simulink model "Hardmon_Model"  (R2023b)
settings: Solver=FixedStepDiscrete  StartTime=0.0  StopTime=10  RelTol=1e-3
libraries: msbUtilities x1
settings Model: Creator=heyka  LastModifiedBy=nickj
settings DataIOCC: ExternalInput=test_temp.getElement('Temp 1'),test_temp.getElement('Temp 2')  LoadExternalInput=on
settings OptimizationCC: DefaultParameterBehavior=Inlined  EnhancedBackFolding=on  PassReuseOutputArgsAs=Individual arguments  ZeroExternalMemoryAtStartup=off  ZeroInternalMemoryAtStartup=off  OptimizeBlockOrder=speed  DifferentSizesBufferReuse=on  OptimizationCustomize=off  EfficientTunableParamExpr=on
settings DebuggingCC: SolverPrmCheckMsg=warning  ParameterTunabilityLossMsg=error  StateNameClashWarn=warning
settings HardwareCC: ProdBitPerInt=16  ProdBitPerPointer=16  ProdBitPerSizeT=16  ProdBitPerPtrDiffT=16  ProdLargestAtomicFloat=None  ProdWordSize=16  ProdHWDeviceType=STMicroelectronics->ST10/Super10
settings SFSimCC: MATLABDynamicMemAlloc=off  SimTargetLang=C++
settings RTWCC: Description=Embedded Coder  SystemTargetFile=ert.tlc  GenCodeOnly=on  TemplateMakefile=ert_default_tmf  Toolchain=MinGW64 | gmake (64-bit Windows)  BuildConfiguration=Faster Runs  PortableWordSizes=on  DataTypeReplacement=CDataTypesFixedWidth  TargetLang=C++
settings CodeAppCC: ForceParamTrailComments=on  IgnoreCustomStorageClasses=off  OperatorAnnotations=on  SimulinkDataObjDesc=on  SFDataObjDesc=on  MATLABFcnDesc=on  InsertBlockDesc=on  StateflowObjectComments=on  InlinedPrmAccess=Macros
settings ERTTargetCC: TargetLangStandard=C++11 (ISO)  GenerateSampleERTMain=on  CodeInterfacePackaging=C++ class  SupportNonFinite=off  SupportComplex=off  CastingMode=Standards  ArrayLayout=Row-major  InlinedParameterPlacement=NonHierarchical  RootIOFormat=Structure reference  ERTCustomFileTemplate=example_file_process.tlc  ERTFilePackagingFormat=Compact  SuppressUnreachableDefaultCases=off  IndentSize=4  MaxIdInt64=INT64_MAX  MinIdInt64=INT64_MIN  MaxIdUint64=UINT64_MAX  MaxIdInt32=INT32_MAX  MinIdInt32=INT32_MIN  MaxIdUint32=UINT32_MAX  MaxIdInt16=INT16_MAX  MinIdInt16=INT16_MIN  MaxIdUint16=UINT16_MAX  MaxIdInt8=INT8_MAX  MinIdInt8=INT8_MIN  MaxIdUint8=UINT8_MAX

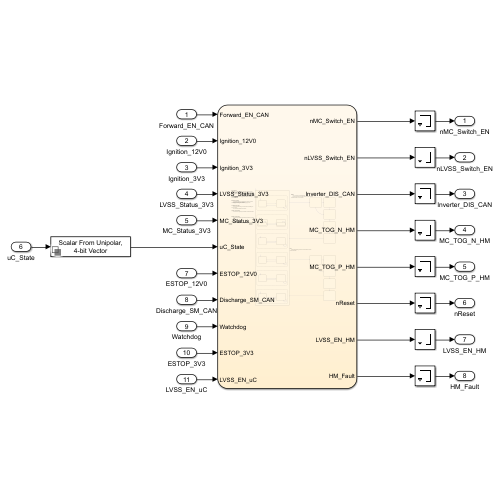
[thumbnail: Simulink's stored preview of the top-level diagram]
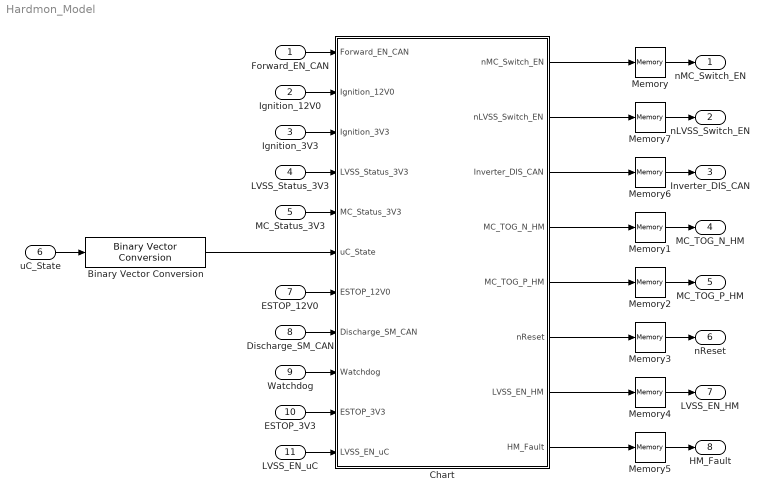
== system Hardmon_Model ==
  Forward_EN_CAN : Inport  OutDataTypeStr=boolean
  Ignition_12V0 : Inport  Port=2  OutDataTypeStr=boolean
  Ignition_3V3 : Inport  Port=3  OutDataTypeStr=boolean
  LVSS_Status_3V3 : Inport  Port=4  OutDataTypeStr=boolean
  MC_Status_3V3 : Inport  Port=5  OutDataTypeStr=boolean
  uC_State : Inport  Port=6  OutDataTypeStr=uint8  PortDimensions=4
  ESTOP_12V0 : Inport  Port=7  OutDataTypeStr=boolean
  Discharge_SM_CAN : Inport  Port=8  OutDataTypeStr=uint8
  Watchdog : Inport  Port=9  OutDataTypeStr=boolean
  ESTOP_3V3 : Inport  Port=10  OutDataTypeStr=boolean
  LVSS_EN_uC : Inport  Port=11  OutDataTypeStr=boolean
  Binary Vector Conversion : msbUtilities/Binary Vector Conversion  LabelModeActiveChoice=From Unipolar  Convert=Binary-coded vector to scalar  Encoding=Unipolar (magnitude)  InputLength=4  InputReverse=LSB at index 1  OutputLength=4  OutputReverse=LSB at index 1  DataType=uint8
  Chart : Stateflow chart  TreatAsAtomicUnit=on
      settings: PortSchema="{\"entries\":[{\"content\":{\"sides\":[{\"content\":{\"connectorIds\":[\"In1\",\"In2\",\"In3\",\"In4\",\"In5\",\"In6\",\"In7\",\"In8\",\"In9\",\"In10\",\"In11\"]},\"type\":\"ConnectorPlacement.EquallySpacedRectSide\",\"uuid\":\"6d1a41ef-67e8-41d6-9adb-1761831f6d0e\"},{\"content\":{\"connectorIds\":[\"Out1\",\"Out8\",\"Out2\",\"Out3\",\"Out4\",\"Out5\",\"Out6\",\"Out7\"],\"side\":\"RIGHT\"},\"type\":\"ConnectorPlacement.EquallySpacedRectSide\",\"uuid\":\"1c1f5b1f-9a19-48ee-ac61-8a13c1cfd4a8\"},{\"content\":{\"side\":\"TOP\"},\"type\":\"ConnectorPlacement.EquallySpacedRectSide\",\"uuid\":\"7f8ec887-50f7-4fb3-9eed-5aef04cf2afb\"}]},\"type\":\"ConnectorPlacement.EquallySpacedConnector\",\"uuid\":\"822c8876-1e52-4482-83f3-7114ae95ed93\"}],\"packageUris\":[\"http://schema.mathworks.com/mf0/Connector/R2020b\"],\"version\":\"1.0\"}"
  Memory{,1..7} (8 alike) : Memory
  nMC_Switch_EN : Outport  OutDataTypeStr=boolean
  nLVSS_Switch_EN : Outport  Port=2  OutDataTypeStr=boolean
  Inverter_DIS_CAN : Outport  Port=3  OutDataTypeStr=boolean
  MC_TOG_N_HM : Outport  Port=4  OutDataTypeStr=boolean
  MC_TOG_P_HM : Outport  Port=5  OutDataTypeStr=boolean
  nReset : Outport  Port=6  OutDataTypeStr=boolean
  LVSS_EN_HM : Outport  Port=7  OutDataTypeStr=boolean
  HM_Fault : Outport  Port=8  OutDataTypeStr=boolean
  wires:
  Chart/7(HM_Fault) -> Memory5/1
  uC_State/1 -> Binary Vector Conversion/1
  Forward_EN_CAN/1 -> Chart/1(Forward_EN_CAN)
  Binary Vector Conversion/1 -> Chart/6(uC_State)
  LVSS_Status_3V3/1 -> Chart/4(LVSS_Status_3V3)
  Chart/6(LVSS_EN_HM) -> Memory4/1
  Ignition_12V0/1 -> Chart/2(Ignition_12V0)
  Ignition_3V3/1 -> Chart/3(Ignition_3V3)
  MC_Status_3V3/1 -> Chart/5(MC_Status_3V3)
  ESTOP_12V0/1 -> Chart/7(ESTOP_12V0)
  Discharge_SM_CAN/1 -> Chart/8(Discharge_SM_CAN)
  Watchdog/1 -> Chart/9(Watchdog)
  ESTOP_3V3/1 -> Chart/10(ESTOP_3V3)
  LVSS_EN_uC/1 -> Chart/11(LVSS_EN_uC)
  Chart/1(nMC_Switch_EN) -> Memory/1
  Chart/2(Inverter_DIS_CAN) -> Memory6/1
  Chart/3(MC_TOG_N_HM) -> Memory1/1
  Chart/4(MC_TOG_P_HM) -> Memory2/1
  Memory/1 -> nMC_Switch_EN/1
  Chart/5(nReset) -> Memory3/1
  Memory6/1 -> Inverter_DIS_CAN/1
  Memory1/1 -> MC_TOG_N_HM/1
  Memory2/1 -> MC_TOG_P_HM/1
  Memory3/1 -> nReset/1
  Memory4/1 -> LVSS_EN_HM/1
  Memory5/1 -> HM_Fault/1
  Memory7/1 -> nLVSS_Switch_EN/1
  Chart/8(nLVSS_Switch_EN) -> Memory7/1

== stateflow chart Hardmon_Model/Chart ==
  note: General Notes:
      | - LVSS_EN_HM = LVSS_EN_uC is used to ensure that if the HardMon triggers
      | - No transitions occur when the uC_State is 6 or 7 to ensure that nothing tranistions when the motor controller is already discharging
  state Normal_Operation
    state ESTOP_Checking [parallel]
      settings: executionOrder=1
      state count
        entry:
        ESTOP_Counter = ESTOP_Counter + 1;
      state ESTOP_Inactive
        entry:
        HM_Fault = false;
        ESTOP_Counter = 0;
        nMC_Switch_EN = false;
        nLVSS_Switch_EN = false;
        LVSS_EN_HM = LVSS_EN_uC;
      (default) -> ESTOP_Inactive
      ESTOP_Inactive -> Normal_Operation.ESTOP_Checking.count : [ESTOP_3V3 == true && uC_State ~= 7 && uC_State ~= 6 ]
      Normal_Operation.ESTOP_Checking.count -> ESTOP_Inactive [order 2] : [ESTOP_3V3 == true || uC_State == 7 || uC_State == 6 ]
      Normal_Operation.ESTOP_Checking.count -> Normal_Operation.ESTOP_Checking.count [order 1] : after(0.1,sec)
    state Watchdog_Checking [parallel]
      settings: executionOrder=2
      state WD_Low
        entry:
        WD_Counter = 0;
        state Counting
          entry:
          WD_Counter = WD_Counter + 1;
        Normal_Operation.Watchdog_Checking.WD_Low.Counting -> Normal_Operation.Watchdog_Checking.WD_Low.Counting [order 2] : after(0.5, sec)
      state WD_High
        entry:
        WD_Counter = 0;
        state Counting
          entry:
          WD_Counter = WD_Counter + 1;
        Normal_Operation.Watchdog_Checking.WD_High.Counting -> Normal_Operation.Watchdog_Checking.WD_High.Counting [order 2] : after(0.5, sec)
      (default) -> WD_Low
      Normal_Operation.Watchdog_Checking.WD_Low.Counting -> WD_High [order 1] : [Watchdog == true]
      Normal_Operation.Watchdog_Checking.WD_High.Counting -> WD_Low [order 1] : [Watchdog == false]
    state Invalid_State_Checking [parallel]
      settings: executionOrder=3
      state count
        entry:
        Invalid_State_Counter = Invalid_State_Counter + 1;
      state Invalid_State_Inactive
        entry:
        HM_Fault = false;
        Invalid_State_Counter = 0;
        nMC_Switch_EN = false;
        nLVSS_Switch_EN = false;
        LVSS_EN_HM = LVSS_EN_uC;
      (default) -> Normal_Operation.Invalid_State_Checking.Invalid_State_Inactive
      Normal_Operation.Invalid_State_Checking.Invalid_State_Inactive -> Normal_Operation.Invalid_State_Checking.count : [(Forward_EN_CAN ~= true || Ignition_3V3 ~= true) && uC_State == 3]
      Normal_Operation.Invalid_State_Checking.count -> Normal_Operation.Invalid_State_Checking.Invalid_State_Inactive [order 2] : [~((Forward_EN_CAN ~= true || Ignition_3V3 ~= true) && uC_State == 3)]
      Normal_Operation.Invalid_State_Checking.count -> Normal_Operation.Invalid_State_Checking.count [order 1] : after(0.5,sec)
    state Ignition_Level_Checking [parallel]
      settings: executionOrder=4
      state count
        entry:
        Ignition_State_Counter = Ignition_State_Counter + 1;
      state Ignition_State_Inactive
        entry:
        HM_Fault = false;
        Ignition_State_Counter = 0;
        nMC_Switch_EN = false;
        nLVSS_Switch_EN = false;
        LVSS_EN_HM = LVSS_EN_uC;
      (default) -> Ignition_State_Inactive
      Ignition_State_Inactive -> Normal_Operation.Ignition_Level_Checking.count : [Ignition_3V3 ~= Ignition_12V0  && uC_State ~= 6 ]
      Normal_Operation.Ignition_Level_Checking.count -> Ignition_State_Inactive [order 2] : [Ignition_3V3 == Ignition_12V0  || uC_State == 6 ]
      Normal_Operation.Ignition_Level_Checking.count -> Normal_Operation.Ignition_Level_Checking.count [order 1] : after(0.5,sec)
    state ESTOP_Level_Checking [parallel]
      settings: executionOrder=5
      state count
        entry:
        ESTOP_State_Counter = ESTOP_State_Counter + 1;
      state ESTOP_State_Inactive
        entry:
        HM_Fault = false;
        ESTOP_State_Counter = 0;
        nMC_Switch_EN = false;
        nLVSS_Switch_EN = false;
        LVSS_EN_HM = LVSS_EN_uC;
      (default) -> ESTOP_State_Inactive
      ESTOP_State_Inactive -> Normal_Operation.ESTOP_Level_Checking.count : [ESTOP_3V3 ~= ESTOP_12V0  && uC_State ~= 6 ]
      Normal_Operation.ESTOP_Level_Checking.count -> ESTOP_State_Inactive [order 2] : [ESTOP_3V3 == ESTOP_12V0  || uC_State == 6 ]
      Normal_Operation.ESTOP_Level_Checking.count -> Normal_Operation.ESTOP_Level_Checking.count [order 1] : after(0.5,sec)
    state LVSS_Checking [parallel]
      settings: executionOrder=6
      state count
        entry:
        LVSS_Counter = LVSS_Counter + 1;
      state Invalid_State_Inactive
        entry:
        HM_Fault = false;
        LVSS_Counter = 0;
        nMC_Switch_EN = false;
        nLVSS_Switch_EN = false;
        LVSS_EN_HM = LVSS_EN_uC;
      (default) -> Normal_Operation.LVSS_Checking.Invalid_State_Inactive
      Normal_Operation.LVSS_Checking.Invalid_State_Inactive -> Normal_Operation.LVSS_Checking.count : [LVSS_Status_3V3 ~= LVSS_EN_uC  && uC_State ~= 6 ]
      Normal_Operation.LVSS_Checking.count -> Normal_Operation.LVSS_Checking.Invalid_State_Inactive [order 2] : [LVSS_Status_3V3 == LVSS_EN_uC  || uC_State == 6 ]
      Normal_Operation.LVSS_Checking.count -> Normal_Operation.LVSS_Checking.count [order 1] : after(0.5,sec)
  note: RESET
      | - Only occurs when the watchdog faults
      | - Ensure that the motor controller and lvss is correclty shutdown and holds the MCuC in the reset state
  note: ESTOP Checking:
      | - Checks for ESTOP being triggered but MCUC not entering ESTOP state
  state MC_RESET_INIT
    entry:
    nMC_Switch_EN = true;
    nLVSS_Switch_EN = true;
  state MC_DISCHARGE
    entry:
    HM_Fault = true;
    Inverter_DIS_CAN = true;
  note: Watchdog_Checking
      | - Checks that the MCuC is operational by requiring a constant watchdog gpio to be toggled by the MCuC
      | - Applies a hardware reset instead of triggering a fault
  note: Invalid State Checking
      | - Checks if the MCuC being in the active state is possible given the current inputs
      | - Only valid during the MCuC active state
  state MC_POWERDOWN
    entry:
    nReset = true;
    Inverter_DIS_CAN = false;
    MC_TOG_P_HM = false;
    MC_TOG_N_HM = true;
    exit:
    MC_TOG_P_HM = false;
    MC_TOG_N_HM = false;
  note: Ignition Level Checking
      | - Ensures that the ignition signal matches with both level shifters
  note: ESTOP Level Checking
      | - Ensures that the ESTOP signal matches with both level shifters
  note: LVSS Status Checking
      | - Ensures that the LVSS status matches the LVSS ON command
  state LVSS_Powerdown
    entry:
    LVSS_EN_HM = false;
  state Enter_Fault
    entry:
    nReset = false;
    HM_Fault = true;
    exit:
    nMC_Switch_EN = false;
    nLVSS_Switch_EN = false;
    nReset = true;
  note: Fault
      | - Normal fault handling, ensures the correct shutdown of motor controller and LVSS
  state MC_FAULT_INIT
    entry:
    nMC_Switch_EN = true;
    nLVSS_Switch_EN = true;
  state MC_DISCHARGE_FAULT
    entry:
    HM_Fault = true;
    Inverter_DIS_CAN = true;
  state MC_POWERDOWN1
    entry:
    HM_Fault  = true;
    Inverter_DIS_CAN = false;
    MC_TOG_P_HM = false;
    MC_TOG_N_HM = true;
    exit:
    MC_TOG_P_HM = false;
    MC_TOG_N_HM = false;
  state LVSS_Powerdown1
    entry:
    LVSS_EN_HM = false;
  state End_Powerdown
    entry:
    nMC_Switch_EN = false;
    nLVSS_Switch_EN = false;
    exit:
    HM_Fault = true;
  (default) -> Normal_Operation
  MC_RESET_INIT -> MC_DISCHARGE [order 1] : [uC_State ~= 0 && uC_State ~= 8]
  Normal_Operation -> MC_RESET_INIT [order 1] : [WD_Counter >= 4 && uC_State ~= 8]
  MC_RESET_INIT -> MC_POWERDOWN [order 2] : [uC_State == 0 || uC_State == 8]
  MC_DISCHARGE -> MC_POWERDOWN : [Discharge_SM_CAN == 4]
  MC_POWERDOWN -> LVSS_Powerdown : [MC_Status_3V3 == false]
  LVSS_Powerdown -> Enter_Fault : [LVSS_Status_3V3 == false]
  Enter_Fault -> Normal_Operation : [uC_State == 8]
  Normal_Operation -> MC_FAULT_INIT [order 2] : [Invalid_State_Counter >= 4 || Ignition_State_Counter >= 4 || LVSS_Counter >=4 || ESTOP_Counter >= 4 || ESTOP_State_Counter >= 4]
  MC_FAULT_INIT -> MC_DISCHARGE_FAULT [order 1] : [uC_State ~= 0 && uC_State ~= 8]
  MC_FAULT_INIT -> MC_POWERDOWN1 [order 2] : [uC_State == 0 || uC_State == 8]
  MC_DISCHARGE_FAULT -> MC_POWERDOWN1 : [Discharge_SM_CAN == 4]
  MC_POWERDOWN1 -> LVSS_Powerdown1 : [MC_Status_3V3 == false]
  LVSS_Powerdown1 -> End_Powerdown : [LVSS_Status_3V3 == false]
  End_Powerdown -> Normal_Operation : [uC_State == 6]
  data: WD_Counter local uint8; Forward_EN_CAN input boolean; Ignition_12V0 input boolean; Ignition_3V3 input boolean; LVSS_Status_3V3 input boolean; MC_Status_3V3 input boolean; uC_State input uint8; nMC_Switch_EN output boolean; Inverter_DIS_CAN output boolean; MC_TOG_N_HM output boolean; MC_TOG_P_HM output boolean; nReset output boolean =1; ESTOP_State_Counter local uint8; Ignition_State_Counter local uint8; Invalid_State_Counter local uint8; LVSS_Counter local uint8; LVSS_EN_HM output boolean; ESTOP_12V0 input boolean; Discharge_SM_CAN input uint8; Watchdog input boolean; ESTOP_Counter local uint8; ESTOP_3V3 input boolean =0; HM_Fault output boolean; LVSS_EN_uC input boolean; nLVSS_Switch_EN output boolean
